simulink model "lorenz_0212"  (R2025b)
settings: Solver=ode4  StartTime=0.0  StopTime=100  FixedStep=0.001  RelTol=1e-3
settings Model: Creator=patrick  LastModifiedBy=patrick

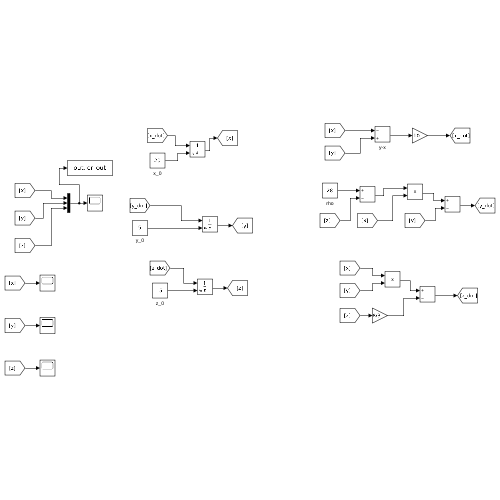
[thumbnail: Simulink's stored preview of the top-level diagram]
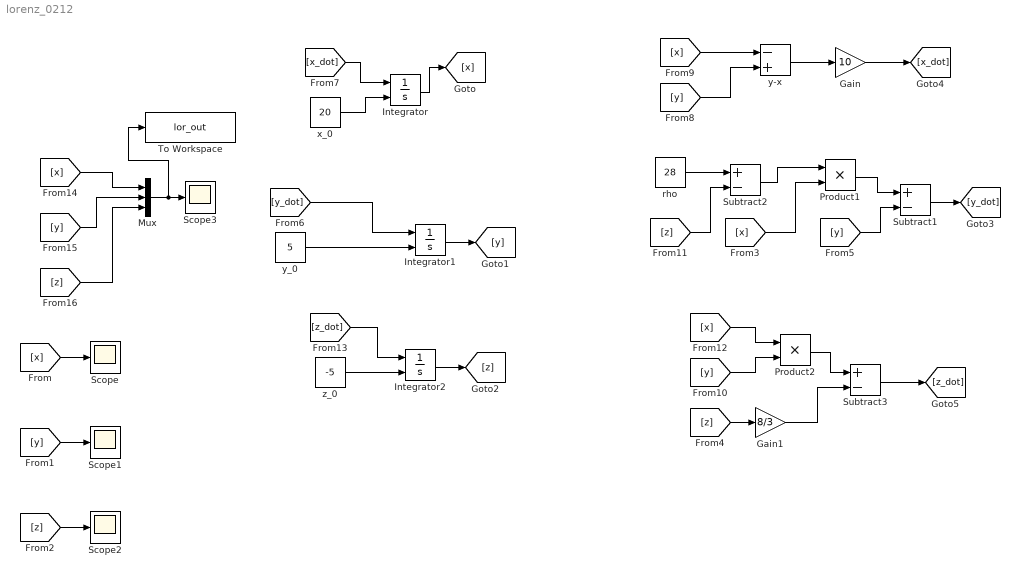
== system lorenz_0212 ==
  Gain : Gain  Gain=10
  Gain1 : Gain  Gain=8/3
  Integrator : Integrator  InitialConditionSource=external
  Integrator1 : Integrator  InitialConditionSource=external
  Integrator2 : Integrator  InitialConditionSource=external
  Mux : Mux  Inputs=3
  Product1 : Product
  Product2 : Product
  Scope{,1..3} (4 alike) : Scope
      Scope settings: ActiveDisplayYMinimum=-1  ActiveDisplayYMaximum=1
      Scope1 settings: ActiveDisplayYMinimum=-1  ActiveDisplayYMaximum=1
      Scope2 settings: ActiveDisplayYMinimum=-1  ActiveDisplayYMaximum=1  DataLoggingVariableName=ScopeData2
      Scope3 settings: ActiveDisplayYMinimum=-33.882427515740019  ActiveDisplayYMaximum=63.571465098155564  DataLoggingVariableName=ScopeData3
  Subtract1 : Sum  Inputs=+-
  Subtract2 : Sum  Inputs=+-
  Subtract3 : Sum  Inputs=+-
  To Workspace : ToWorkspace  VariableName=lor_out  SampleTime=-1
  rho : Constant  Value=28
  x_0 : Constant  Value=20
  y-x : Sum  Inputs=-+
  y_0 : Constant  Value=5
  z_0 : Constant  Value=-5
  wires:
  x_0/1 -> Integrator/2
  Integrator/1 -> [x]
  y_0/1 -> Integrator1/2
  z_0/1 -> Integrator2/2
  y-x/1 -> Gain/1
  Integrator1/1 -> [y]
  [x] -> Scope/1
  [y] -> Scope1/1
  [z] -> Scope2/1
  Subtract1/1 -> [y_dot]
  [y_dot] -> Integrator1/1
  [x_dot] -> Integrator/1
  [y] -> y-x/2
  Gain/1 -> [x_dot]
  [x] -> y-x/1
  [z] -> Gain1/1
  rho/1 -> Subtract2/1
  [z] -> Subtract2/2
  [x] -> Product1/2
  Subtract2/1 -> Product1/1
  Product1/1 -> Subtract1/1
  [y] -> Subtract1/2
  [x] -> Product2/1
  [y] -> Product2/2
  Product2/1 -> Subtract3/1
  Gain1/1 -> Subtract3/2
  [z_dot] -> Integrator2/1
  Integrator2/1 -> [z]
  Subtract3/1 -> [z_dot]
  [z] -> Mux/3
  [y] -> Mux/2
  [x] -> Mux/1
  Mux/1 -> To Workspace/1, Scope3/1
